simulink model "reg_dob"  (R2015b)
settings: Solver=ode45  StartTime=0.0  StopTime=10  RelTol=1e-3
values from neighbouring files (symbols this model uses):
  A = [0 1 0; -4 -.4 40; 0 0 -4]    [hw8.m]
  B = [0;0;2]    [hw8.m]
  C = [1 0 0]    [hw8.m]
  K = place(phi, gamma, zPoles)    [hw8.m]
  L = (place(phi',C',zoPoles))'    [hw8.m]
  T = min(pi/beta_max,Ts/(20*n))    [hw8.m]
  x0 = [0.34;0;0]    [hw8.m]
undefined symbols (not defined in the file or in its folder): gamma, phi
settings Model: Creator=rjv  LastModifiedBy=rjv
settings DataIOCC: SaveFormat=Array
settings DebuggingCC: AllowSymbolicDim=on
settings HardwareCC: ProdBitPerPointer=32  ProdLargestAtomicFloat=None  ProdIntDivRoundTo=Undefined  ProdEndianess=Unspecified  ProdWordSize=32  ProdHWDeviceType=32-bit Generic
settings GRTTargetCC: GeneratePreprocessorConditionals=Disable all
settings ConfigComp: CovModelRefEnable=Off

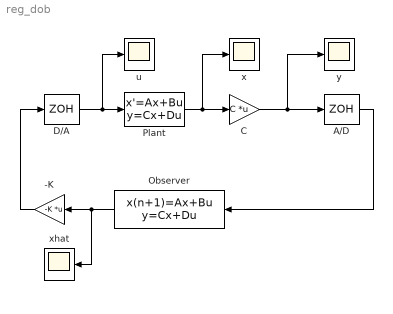
== system reg_dob ==
  -K : Gain  Gain=-K  Multiplication=Matrix(K*u)
  A/D : ZeroOrderHold  SampleTime=T
  C : Gain  Gain=C  Multiplication=Matrix(K*u)
  D/A : ZeroOrderHold  SampleTime=T
  Observer : DiscreteStateSpace  A=phi-gamma*K-L*C  B=L  C=eye(length(A))  D=zeros(length(A),min(size((C))))  X0=C'/(C*C')*C*x0  SampleTime=T
  Plant : StateSpace  A=A  B=B  C=eye(length(A))  D=zeros(length(A),min(size((B))))  X0=x0
  u : Scope
  x : Scope
  xhat : Scope
  y : Scope
  wires:
  Plant/1 -> x/1, C/1
  D/A/1 -> u/1, Plant/1
  C/1 -> y/1, A/D/1
  A/D/1 -> Observer/1
  Observer/1 -> xhat/1, -K/1
  -K/1 -> D/A/1
